simulink model "awgnmodel"  (R2018a)
settings: Solver=VariableStepAuto  StartTime=0.0  StopTime=Simulationtime  RelTol=1e-3
libraries: commutil2 x4, commsink2 x2, commfilt2 x2, commdigbbndpm3 x2, commchan3 x1, commrandsrc3 x1
settings Model: Creator=sdf  LastModifiedBy=sdf

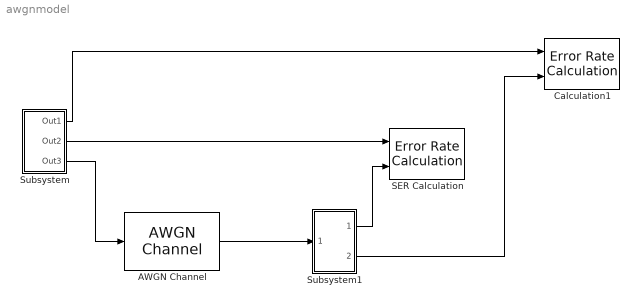
== system awgnmodel ==
  " Calculation1" : commsink2/Error Rate Calculation  N=0  st_delay=0  cp_mode=Entire frame  subframe=[]  PMode=Workspace  WsName=BER  RsMode2=off  stop=off  numErr=100  maxBits=1e6
  AWGN Channel : commchan3/AWGN Channel  InputProcessing=Columns as channels (frame based)  seed=123456  noiseMode="Signal to noise ratio  (SNR)"  EbNodB=10  EsNodB=10  SNRdB=SNR  bitsPerSym=1  Ps=1  Tsym=1  variance=1
  SER Calculation : commsink2/Error Rate Calculation  N=0  st_delay=0  cp_mode=Entire frame  subframe=[]  PMode=Workspace  WsName=SER  RsMode2=off  stop=off  numErr=100  maxBits=1e6
  Subsystem : Subsystem
  Subsystem1 : Subsystem
  wires:
  AWGN Channel/1 -> Subsystem1/1(In1)
  Subsystem1/1(Out1) -> SER Calculation/2
  Subsystem1/2(Out2) -> " Calculation1"/2
  Subsystem/1(Out1) -> " Calculation1"/1
  Subsystem/2(Out2) -> SER Calculation/1
  Subsystem/3(Out3) -> AWGN Channel/1

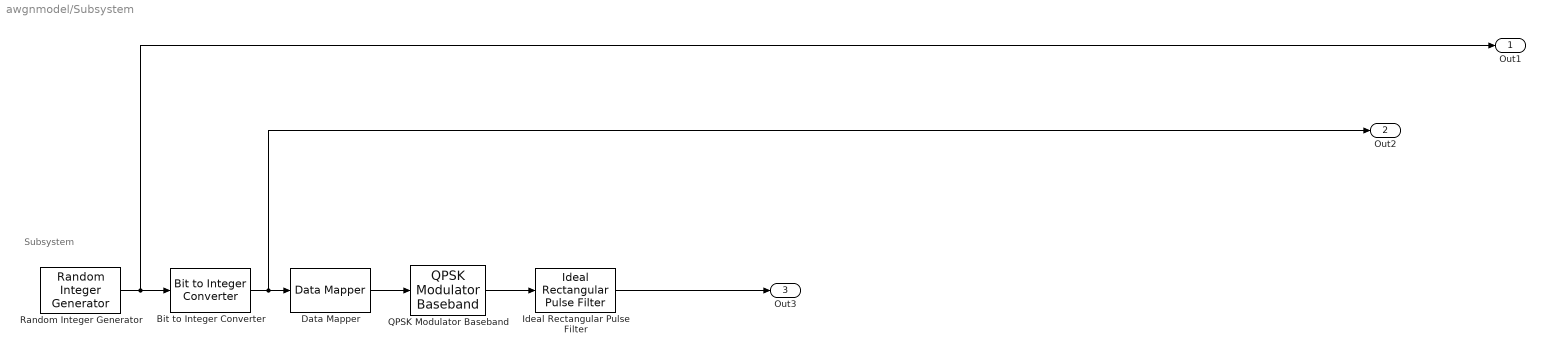
== system awgnmodel/Subsystem ==
  note: Subsystem
  Bit to Integer Converter : commutil2/Bit to Integer Converter  nbits=2  bitOrder=MSB first  signedOutputValues=Unsigned  outDtype=Inherit via internal rule  outDtypeSigned=Inherit via internal rule
  Data Mapper : commutil2/Data Mapper  MapMode=Binary to Gray  M=4  MapVec=[0 1 3 2 7 6 4 5]
      settings: SourceProductName=Communications System Toolbox  SourceProductBaseCode=CM
  Ideal Rectangular Pulse Filter : commfilt2/Ideal Rectangular Pulse Filter  pulseLen=8  pulseDelay=0  InputProcessing=Columns as channels (frame based)  RateOptions=Enforce single-rate processing  sampMode=Mute  normCheck=off  normMode=Sum of samples  filterGain=1  saveAsFlag=0  roundingMode=Floor  overflowMode=off  firstCoeffDataTypeStr=Inherit: Same word length as input  firstCoeffMin=[]  firstCoeffMax=[]  firstCoeffLastDataTypeStr=Inherit: Same word length as input  outputDataTypeStr=Inherit: Same as accumulator  outputMin=[]  outputMax=[]  outputLastDataTypeStr=Inherit: Same as accumulator
      settings: SourceProductName=Communications System Toolbox  SourceProductBaseCode=CM
  QPSK Modulator Baseband : commdigbbndpm3/QPSK Modulator Baseband  InType=Integer  Enc=Gray  Ph=pi/4  outDtype=double  outWordLen=16  outUDDataType=sfix(16)  outFracLenMode=Best precision  outFracLen=15  outDataTypeStr=double  outLastDataTypeStr=double
  Random Integer Generator : commrandsrc3/Random Integer Generator  SetSize=2  SeedSource=Parameter  Seed=37  SampleTime=1/400000  SamplesPerFrame=400000  OutputDataType=double  SimulateUsing=Interpreted execution
  Out1 : Outport
  Out2 : Outport  Port=2
  Out3 : Outport  Port=3
  wires:
  Data Mapper/1 -> QPSK Modulator Baseband/1
  Random Integer Generator/1 -> Out1/1, Bit to Integer Converter/1
  Ideal Rectangular Pulse Filter/1 -> Out3/1
  QPSK Modulator Baseband/1 -> Ideal Rectangular Pulse Filter/1
  Bit to Integer Converter/1 -> Out2/1, Data Mapper/1

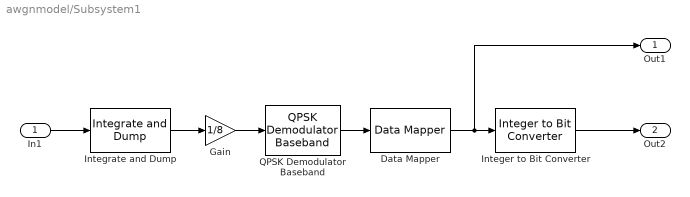
== system awgnmodel/Subsystem1 ==
  In1 : Inport
  Data Mapper : commutil2/Data Mapper  MapMode=Binary to Gray  M=4  MapVec=[0 1 3 2 7 6 4 5]
      settings: SourceProductName=Communications System Toolbox  SourceProductBaseCode=CM
  Gain : Gain  Gain=1/8
  Integer to Bit Converter : commutil2/Integer to Bit Converter  nbits=2  signedInputValues=Unsigned  bitOrder=MSB first  outDtype=Inherit via internal rule
  Integrate and Dump : commfilt2/Integrate and Dump  obssamples=8  offsetsamples=0  nodump=off  roundingMode=Floor  overflowMode=off  outputDataTypeStr=Inherit: Same as accumulator  outputLastDataTypeStr=Inherit: Same as accumulator
      settings: SourceProductName=Communications System Toolbox
  QPSK Demodulator Baseband : commdigbbndpm3/QPSK Demodulator Baseband  OutType=Integer  DecType=Hard decision  VarSource=Dialog  Variance=1  Dec=Gray  Ph=pi/4  outDtype1=Inherit via internal rule  outDtype2=Inherit via internal rule  derotateFactorWordLen=16  derotateFactorDataTypeStr=Inherit: Same word length as input  derotateFactorLastDataTypeStr=Inherit: Same word length as input
  Out1 : Outport
  Out2 : Outport  Port=2
  wires:
  In1/1 -> Integrate and Dump/1
  Data Mapper/1 -> Out1/1, Integer to Bit Converter/1
  Gain/1 -> QPSK Demodulator Baseband/1
  Integrate and Dump/1 -> Gain/1
  Integer to Bit Converter/1 -> Out2/1
  QPSK Demodulator Baseband/1 -> Data Mapper/1
